simulink model "mutifreqsinewave"  (R2020b)
settings: Solver=VariableStepAuto  StartTime=0.0  StopTime=0.3  RelTol=1e-3
settings Model: Creator=E0149968  LastModifiedBy=E0149968

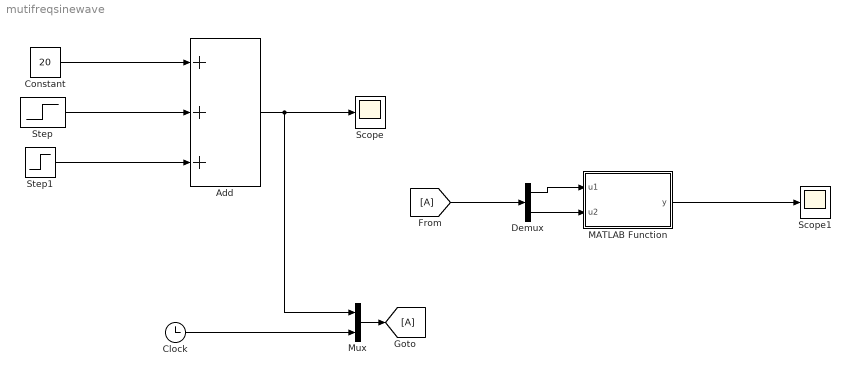
== system mutifreqsinewave ==
  Add : Sum  Inputs=+++
  Clock : Clock
  Constant : Constant  Value=20  SampleTime=1e-6
  Demux : Demux  Outputs=2
  MATLAB Function : MATLAB Function  TreatAsAtomicUnit=on
  Mux : Mux  Inputs=2
  Scope : Scope
  Scope1 : Scope
  Step : Step  Time=0.1  After=20  SampleTime=1e-6
  Step1 : Step  Time=0.2  After=20  SampleTime=1e-6
  wires:
  Constant/1 -> Add/1
  Step/1 -> Add/2
  Step1/1 -> Add/3
  Add/1 -> Mux/1, Scope/1
  Clock/1 -> Mux/2
  Demux/1 -> MATLAB Function/1(u1)
  Demux/2 -> MATLAB Function/2(u2)
  Mux/1 -> [A]
  [A] -> Demux/1
  MATLAB Function/1(y) -> Scope1/1

== matlab function mutifreqsinewave/MATLAB Function ==
  data: u1 input; y output; u2 input
function y = fcn(u1,u2)

y = sin(2*pi*u1*u2);
end
